simulink model "Lab2_P2Q2"  (R2019a)
settings: Solver=FixedStepDiscrete  StartTime=0.0  StopTime=10.0  FixedStep=0.01  RelTol=1e-3
settings Model: Creator=Kyle Bremner  LastModifiedBy=keeshigan

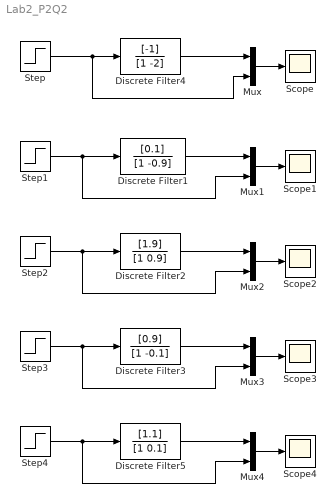
== system Lab2_P2Q2 ==
  Discrete Filter1 : DiscreteFilter  Numerator=[0.1]  Denominator=[1 -0.9]  FilterStructure=Direct form I
  Discrete Filter2 : DiscreteFilter  Numerator=[1.9]  Denominator=[1 0.9]  FilterStructure=Direct form I
  Discrete Filter3 : DiscreteFilter  Numerator=[0.9]  Denominator=[1 -0.1]  FilterStructure=Direct form I
  Discrete Filter4 : DiscreteFilter  Numerator=[-1]  Denominator=[1 -2]  FilterStructure=Direct form I
  Discrete Filter5 : DiscreteFilter  Numerator=[1.1]  Denominator=[1 0.1]  FilterStructure=Direct form I
  Mux{,1..4} (5 alike) : Mux  Inputs=2
  Scope{,1..4} (5 alike) : Scope
  Step{,1..4} (5 alike) : Step  SampleTime=0
  wires:
  Mux/1 -> Scope/1
  Discrete Filter1/1 -> Mux1/1
  Step1/1 -> Mux1/2, Discrete Filter1/1
  Discrete Filter2/1 -> Mux2/1
  Step2/1 -> Mux2/2, Discrete Filter2/1
  Discrete Filter3/1 -> Mux3/1
  Step3/1 -> Mux3/2, Discrete Filter3/1
  Discrete Filter5/1 -> Mux4/1
  Step4/1 -> Mux4/2, Discrete Filter5/1
  Step/1 -> Mux/2, Discrete Filter4/1
  Discrete Filter4/1 -> Mux/1
  Mux1/1 -> Scope1/1
  Mux2/1 -> Scope2/1
  Mux3/1 -> Scope3/1
  Mux4/1 -> Scope4/1
